simulink model "A1_s203658_Trosborg_s203678_Hansen_s203679_Fertin"  (R2023b)
settings: Solver=VariableStepAuto  StartTime=0  StopTime=10860  MaxStep=0.1  RelTol=1e-3
model workspace: external: MAT-File data_workspace.mat (data not in the file)
undefined symbols (not defined in the file or in its folder): Ccell, Cth, NumCellsParallel, Rth, Tcell0
libraries: simulink x13
(part 2 of 2)

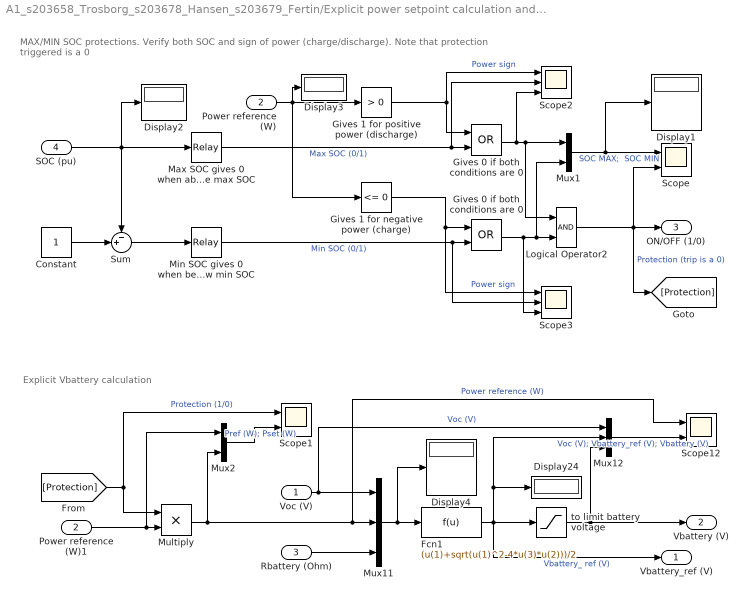
== system A1_s203658_Trosborg_s203678_Hansen_s203679_Fertin/Explicit power setpoint calculation and SOC protection2 ==
  note: Explicit Vbattery calculation
  note: MAX/MIN SOC protections. Verify both SOC and sign of power (charge/discharge). Note that protection triggered is a 0
  Voc (V) : Inport
  Power reference (W) : Inport  Port=2
  Rbattery (Ohm) : Inport  Port=3
  SOC (pu) : Inport  Port=4
  Constant : Constant
  Display{1..4,24} (5 alike) : Display
  Fcn1 : Fcn  Expr=(u(1)+sqrt(u(1)^2-4*u(3)*u(2)))/2
  "Gives 0 if both conditions are 0 " : Logic  Operator=OR  AllPortsSameDT=off  OutDataTypeStr=boolean
  "Gives 0 if both conditions are 0 " : Logic  Operator=OR  AllPortsSameDT=off  OutDataTypeStr=boolean
  Gives 1 for negative power (charge) : simulink/Logic and Bit Operations/Compare To Zero  relop=<=  OutDataTypeStr=boolean
  Gives 1 for positive power (discharge) : simulink/Logic and Bit Operations/Compare To Zero  relop=>  OutDataTypeStr=boolean
  Logical Operator2 : Logic  AllPortsSameDT=off  OutDataTypeStr=boolean
  "Max SOC gives 0 when above max SOC " : Relay  OnSwitchValue=SOC_Max  OffSwitchValue=SOC_Max - 1.8e-7  OnOutputValue=0  OffOutputValue=1
  Min SOC gives 0 when below min SOC : Relay  OnSwitchValue=1-SOC_Min  OffSwitchValue=1-(SOC_Min+1.8e-7)  OnOutputValue=0  OffOutputValue=1
  Multiply : Product
  Mux1 : Mux  Inputs=2
  Mux11 : Mux  Inputs=3
  Mux12 : Mux  Inputs=3
  Mux2 : Mux  Inputs=2
  Power reference (W)1 : InportShadow  Port=2
  Scope : Scope  NumInputPorts=2
  Scope1 : Scope  NumInputPorts=2
  Scope12 : Scope  NumInputPorts=2
  Scope2 : Scope  NumInputPorts=3
  Scope3 : Scope  NumInputPorts=3
  Sum : Sum  Inputs=-+|
  to limit battery voltage : Saturate  UpperLimit=CellVoltage_Max*NumCellsSeries  LowerLimit=CellVoltage_Min*NumCellsSeries
  Vbattery_ref (V) : Outport  VectorParamsAs1DForOutWhenUnconnected=off
  Vbattery (V) : Outport  Port=2  VectorParamsAs1DForOutWhenUnconnected=off
  ON/OFF (1/0) : Outport  Port=3  VectorParamsAs1DForOutWhenUnconnected=off
  wires:
  Voc (V)/1 -> Mux12/1, Mux11/1  "Voc (V)"
  Fcn1/1 -> Vbattery_ref (V)/1, Mux12/2, Display24/1, to limit battery voltage/1  "Vbattery_ ref (V)"
  Mux11/1 -> Display4/1, Fcn1/1
  Mux12/1 -> Scope12/2  "Voc (V); Vbattery_ref (V); Vbattery (V)"
  Constant/1 -> Sum/2
  SOC (pu)/1 -> Display2/1, Sum/1, "Max SOC gives 0 when above max SOC "/1
  Sum/1 -> Min SOC gives 0 when below min SOC/1
  Gives 1 for negative power (charge)/1 -> "Gives 0 if both conditions are 0 "/1, Scope3/1  "Power sign"
  Gives 1 for positive power (discharge)/1 -> "Gives 0 if both conditions are 0 "/1, Scope2/1  "Power sign"
  Power reference (W)/1 -> Gives 1 for positive power (discharge)/1, Gives 1 for negative power (charge)/1, Display3/1
  "Gives 0 if both conditions are 0 "/1 -> Mux1/1, Logical Operator2/1, Scope2/3
  "Gives 0 if both conditions are 0 "/1 -> Mux1/2, Logical Operator2/2, Scope3/3
  Logical Operator2/1 -> [Protection], ON/OFF (1/0)/1, Scope/2  "Protection (trip is a 0)"
  Mux1/1 -> Display1/1, Scope/1  "SOC MAX;  SOC MIN"
  Power reference (W)1/1 -> Mux2/1, Multiply/2
  [Protection] -> Scope1/1, Multiply/1  "Protection (1/0)"
  Multiply/1 -> Mux2/2, Scope12/1, Mux11/2  "Power reference (W)"
  Rbattery (Ohm)/1 -> Mux11/3
  Mux2/1 -> Scope1/2  "Pref (W); Pset (W)"
  Min SOC gives 0 when below min SOC/1 -> Scope3/2, "Gives 0 if both conditions are 0 "/2  "Min SOC (0/1)"
  to limit battery voltage/1 -> Vbattery (V)/1, Mux12/3
  "Max SOC gives 0 when above max SOC "/1 -> Scope2/2, "Gives 0 if both conditions are 0 "/2  "Max SOC (0/1)"

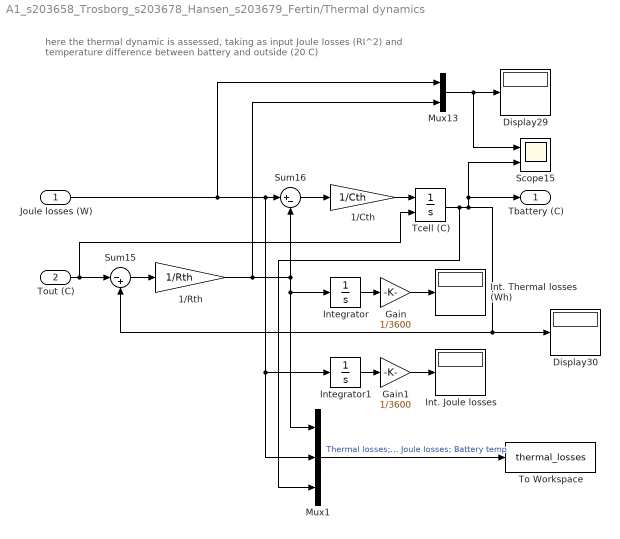
== system A1_s203658_Trosborg_s203678_Hansen_s203679_Fertin/Thermal dynamics ==
  note: here the thermal dynamic is assessed, taking as input Joule losses (RI^2)
      | and temperature difference between battery and outside (20 C)
  Joule losses (W) : Inport
  Tout (C) : Inport  Port=2
  1/Cth : Gain  Gain=1/Cth
  1/Rth : Gain  Gain=1/Rth
  Display29 : Display
  Display30 : Display
  Gain : Gain  Gain=1/3600
  Gain1 : Gain  Gain=1/3600
  Int. Joule losses : Display
  Int. Thermal losses (Wh) : Display
  Integrator : Integrator
  Integrator1 : Integrator
  Mux1 : Mux  Inputs=3
  Mux13 : Mux  Inputs=2
  Scope15 : Scope  NumInputPorts=2
  Sum15 : Sum  Inputs=|-+
  Sum16 : Sum  Inputs=|+-
  Tcell (C) : Integrator  InitialConditionSource=external  InitialCondition=Tcell0  ZeroCross=off
  To Workspace : ToWorkspace  VariableName=thermal_losses  SaveFormat=Timeseries  SampleTime=-1
  Tbattery (C) : Outport  VectorParamsAs1DForOutWhenUnconnected=off
  wires:
  1/Rth/1 -> Mux1/1, Integrator/1, Sum16/2, Mux13/2
  Joule losses (W)/1 -> Mux13/1, Integrator1/1, Mux1/2, Sum16/1
  Sum16/1 -> 1/Cth/1
  Sum15/1 -> 1/Rth/1
  1/Cth/1 -> Tcell (C)/1
  Mux13/1 -> Display29/1, Scope15/1
  Tcell (C)/1 -> Mux1/3, Tbattery (C)/1, Scope15/2, Sum15/2, Display30/1
  Tout (C)/1 -> Tcell (C)/2, Sum15/1
  Mux1/1 -> To Workspace/1  "Thermal losses; Joule losses; Battery temp"
  Integrator/1 -> Gain/1
  Integrator1/1 -> Gain1/1
  Gain/1 -> Int. Thermal losses (Wh)/1
  Gain1/1 -> Int. Joule losses/1

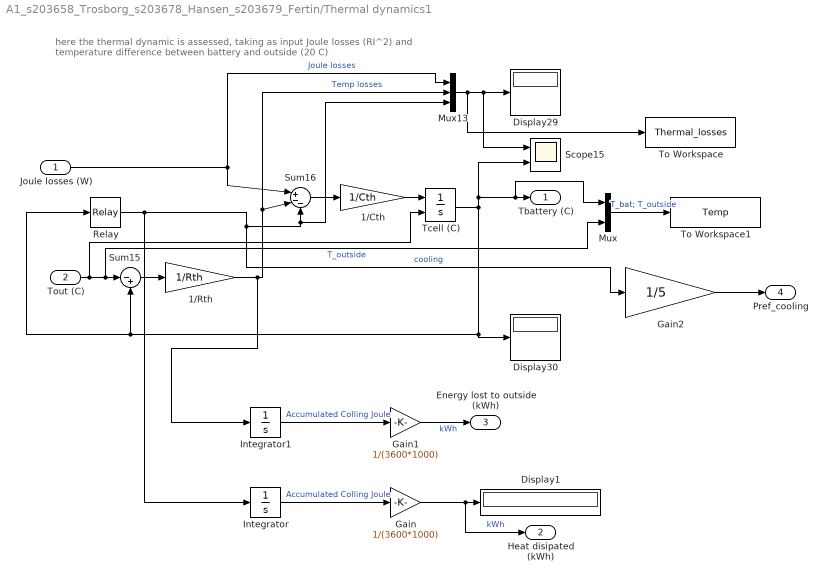
== system A1_s203658_Trosborg_s203678_Hansen_s203679_Fertin/Thermal dynamics1 ==
  note: here the thermal dynamic is assessed, taking as input Joule losses (RI^2)
      | and temperature difference between battery and outside (20 C)
  Joule losses (W) : Inport
  Tout (C) : Inport  Port=2
  1/Cth : Gain  Gain=1/Cth
  1/Rth : Gain  Gain=1/Rth
  Display1 : Display
  Display29 : Display
  Display30 : Display
  Gain : Gain  Gain=1/(3600*1000)
  Gain1 : Gain  Gain=1/(3600*1000)
  Gain2 : Gain  Gain=1/5
  Integrator : Integrator
  Integrator1 : Integrator
  Mux : Mux  Inputs=2
  Mux13 : Mux  Inputs=3
  Relay : Relay  OnSwitchValue=35  OffSwitchValue=25  OnOutputValue=4000
  Scope15 : Scope  NumInputPorts=2
  Sum15 : Sum  Inputs=|-+
  Sum16 : Sum  Inputs=|+--
  Tcell (C) : Integrator  InitialConditionSource=external  InitialCondition=Tcell0  ZeroCross=off
  To Workspace : ToWorkspace  VariableName=Thermal_losses  SaveFormat=Timeseries  SampleTime=-1
  To Workspace1 : ToWorkspace  VariableName=Temp  SaveFormat=Timeseries  SampleTime=-1
  Tbattery (C) : Outport  VectorParamsAs1DForOutWhenUnconnected=off
  Heat disipated (kWh) : Outport  Port=2  VectorParamsAs1DForOutWhenUnconnected=off
  Energy lost to outside (kWh) : Outport  Port=3  VectorParamsAs1DForOutWhenUnconnected=off
  Pref_cooling : Outport  Port=4  VectorParamsAs1DForOutWhenUnconnected=off
  wires:
  Joule losses (W)/1 -> Sum16/1, Mux13/1  "Joule losses"
  Sum16/1 -> 1/Cth/1
  Sum15/1 -> 1/Rth/1
  1/Cth/1 -> Tcell (C)/1
  Mux13/1 -> To Workspace/1, Display29/1, Scope15/1
  Tcell (C)/1 -> Mux/1, Tbattery (C)/1, Scope15/2, Display30/1, Relay/1, Sum15/2
  Tout (C)/1 -> Tcell (C)/2, Mux/2, Sum15/1  "T_outside"
  Integrator/1 -> Gain/1  "Accumulated Colling Joule"
  1/Rth/1 -> Integrator1/1, Sum16/2, Mux13/2  "Temp losses"
  Integrator1/1 -> Gain1/1  "Accumulated Colling Joule"
  Relay/1 -> Gain2/1, Mux13/3, Sum16/3, Integrator/1  "cooling"
  Gain1/1 -> Energy lost to outside (kWh)/1  "kWh"
  Gain/1 -> Heat disipated (kWh)/1, Display1/1  "kWh"
  Mux/1 -> To Workspace1/1  "T_bat; T_outside"
  Gain2/1 -> Pref_cooling/1

== system A1_s203658_Trosborg_s203678_Hansen_s203679_Fertin/Thermal dynamics2 ==
  note: here the thermal dynamic is assessed, taking as input Joule losses (RI^2)
      | and temperature difference between battery and outside (20 C)
  Joule losses (W) : Inport
  Tout (C) : Inport  Port=2
  1/Cth : Gain  Gain=1/Cth
  1/Rth : Gain  Gain=1/Rth
  Display29 : Display
  Display30 : Display
  Mux1 : Mux
  Mux13 : Mux  Inputs=3
  Relay : Relay  OnSwitchValue=35  OffSwitchValue=25  OnOutputValue=4000
  Scope15 : Scope  NumInputPorts=2
  Sum15 : Sum  Inputs=|-+
  Sum16 : Sum  Inputs=|+--
  Tcell (C) : Integrator  InitialConditionSource=external  InitialCondition=Tcell0  ZeroCross=off
  To Workspace : ToWorkspace  VariableName=thermal_losses_trip  SaveFormat=Timeseries  SampleTime=-1
  Tbattery (C) : Outport  VectorParamsAs1DForOutWhenUnconnected=off
  wires:
  1/Rth/1 -> Mux1/1, Sum16/2, Mux13/2  "Temp losses"
  Joule losses (W)/1 -> Mux1/2, Sum16/1, Mux13/1  "Joule losses"
  Sum16/1 -> 1/Cth/1
  Sum15/1 -> 1/Rth/1
  1/Cth/1 -> Tcell (C)/1
  Mux13/1 -> Display29/1, Scope15/1
  Tout (C)/1 -> Tcell (C)/2, Sum15/1
  Relay/1 -> Mux1/4, Mux13/3, Sum16/3  "cooling"
  Tcell (C)/1 -> Tbattery (C)/1, Scope15/2, Display30/1, Mux1/3, Relay/1, Sum15/2
  Mux1/1 -> To Workspace/1  "Thermal losses; Joule losses; Battery temp; Cooling power"
